simulink model "effect_of_controller_on_signal_with_controller"  (R2019a)
settings: Solver=VariableStepAuto  StartTime=0.0  StopTime=10.0  RelTol=1e-3
libraries: dspsrcs4 x1, simulink x1
settings Model: Creator=raxit  LastModifiedBy=raxit

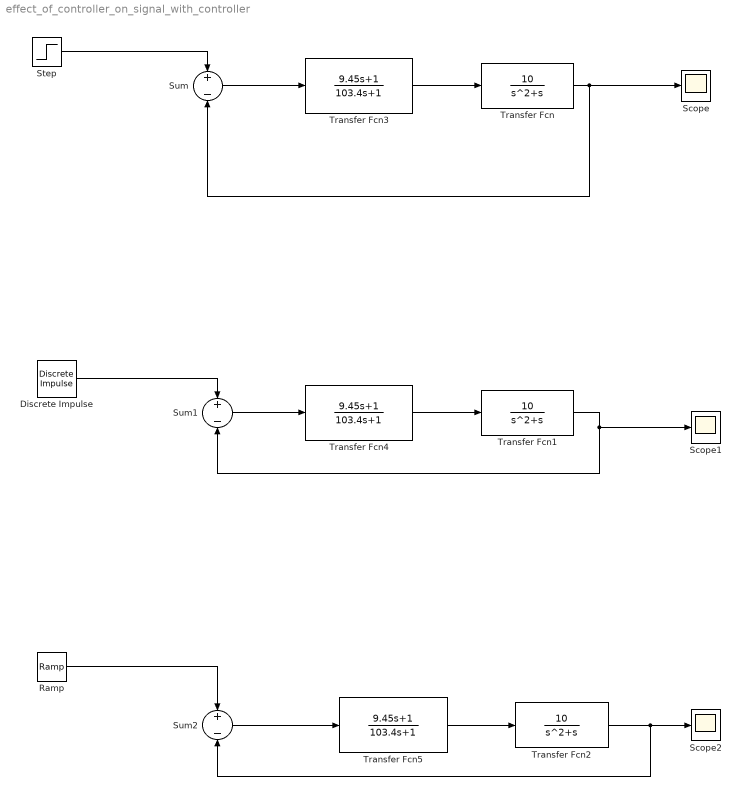
== system effect_of_controller_on_signal_with_controller ==
  Discrete Impulse : dspsrcs4/Discrete  Impulse  Delay=0  SampleTime=1  FrameSample=1  OutputFrames=off  dataType=double  isSigned=on  wordLen=16  udDataType=sfix(16)  fracBitsMode=Best precision  numFracBits=15  OutDataTypeStr=double  LastOutDataTypeStr=double
  Ramp : simulink/Sources/Ramp  slope=1  start=0  InitialOutput=0
  Scope : Scope
  Scope1 : Scope
  Scope2 : Scope
  Step : Step  SampleTime=0
  Sum : Sum  Inputs=+-
  Sum1 : Sum  Inputs=+-
  Sum2 : Sum  Inputs=+-
  Transfer Fcn : TransferFcn  Numerator=[10]  Denominator=[1 1 0]
  Transfer Fcn1 : TransferFcn  Numerator=[10]  Denominator=[1 1 0]
  Transfer Fcn2 : TransferFcn  Numerator=[10]  Denominator=[1 1 0]
  Transfer Fcn3 : TransferFcn  Numerator=[9.45 1]  Denominator=[103.4 1]
  Transfer Fcn4 : TransferFcn  Numerator=[9.45 1]  Denominator=[103.4 1]
  Transfer Fcn5 : TransferFcn  Numerator=[9.45 1]  Denominator=[103.4 1]
  wires:
  Ramp/1 -> Sum2/1
  Sum1/1 -> Transfer Fcn4/1
  Transfer Fcn1/1 -> Scope1/1, Sum1/2
  Discrete Impulse/1 -> Sum1/1
  Step/1 -> Sum/1
  Transfer Fcn/1 -> Scope/1, Sum/2
  Sum/1 -> Transfer Fcn3/1
  Transfer Fcn3/1 -> Transfer Fcn/1
  Transfer Fcn4/1 -> Transfer Fcn1/1
  Transfer Fcn5/1 -> Transfer Fcn2/1
  Sum2/1 -> Transfer Fcn5/1
  Transfer Fcn2/1 -> Scope2/1, Sum2/2
